simulink model "SerialWriteTriggeredSubsystem"  (R2018a)
settings: Solver=FixedStepAuto  StartTime=0.0  StopTime=10.0  FixedStep=.25  RelTol=1e-3  EnableMultiTasking=on
libraries: arduinolib x2
settings Model: ExtModeTrigDuration=2  Creator=jonathancoulter  LastModifiedBy=jonathancoulter
settings OptimizationCC: EnhancedBackFolding=on  PassReuseOutputArgsAs=Individual arguments  MaxStackSize=64  OptimizeBlockOrder=speed  DifferentSizesBufferReuse=on  OptimizationCustomize=off
settings DebuggingCC: ParameterTunabilityLossMsg=error
settings HardwareCC: ProdBitPerInt=16  ProdBitPerPointer=16  ProdBitPerSizeT=16  ProdBitPerPtrDiffT=16  ProdLargestAtomicFloat=None  ProdWordSize=8  ProdHWDeviceType=Atmel->AVR  UseEmbeddedCoderFeatures=off
settings SFSimCC: MATLABDynamicMemAlloc=off
settings RTWCC: SystemTargetFile=ert.tlc  HardwareBoard=Arduino Mega 2560  TLCOptions=-aInlineSetEventsForThisBaseRateFcn=TLC_FALSE -aSuppressMultiTaskScheduler=TLC_FALSE -aRateBasedStepFcn=1  TemplateMakefile=ert_default_tmf  Toolchain=Arduino AVR  BuildConfiguration=Faster Runs  IncludeHyperlinkInReport=on
settings CodeAppCC: ForceParamTrailComments=on  IgnoreCustomStorageClasses=off  OperatorAnnotations=on  SimulinkDataObjDesc=on  SFDataObjDesc=on  InsertBlockDesc=on
settings ERTTargetCC: SupportContinuousTime=on  SupportNonInlinedSFcns=on  SupportVariableSizeSignals=on

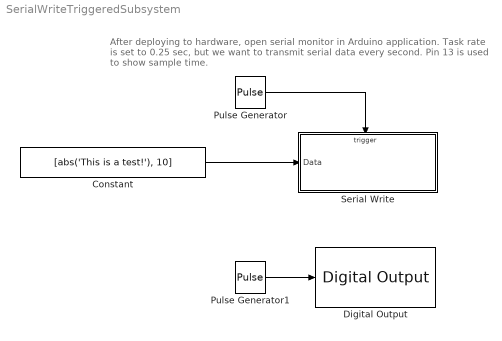
== system SerialWriteTriggeredSubsystem ==
  note: After deploying to hardware, open serial monitor in Arduino application.
      | Task rate is set to 0.25 sec, but we want to transmit serial data every second.
      | Pin 13 is used to show sample time.
  Constant : Constant  Value=[abs('This is a test!'), 10]
  Digital Output : arduinolib/Digital Output  pinNumber=13  blockPlatform=arduino
  Pulse Generator : DiscretePulseGenerator  Period=4  PulseWidth=2  SampleTime=-1
  Pulse Generator1 : DiscretePulseGenerator  SampleTime=-1
  Serial Write : Subsystem
  wires:
  Constant/1 -> Serial Write/1(Data)
  Pulse Generator/1 -> Serial Write/Trigger
  Pulse Generator1/1 -> Digital Output/1

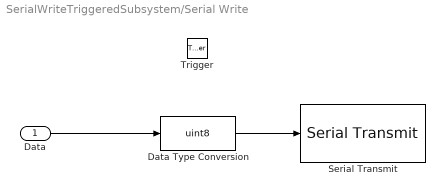
== system SerialWriteTriggeredSubsystem/Serial Write ==
  Data : Inport
  Trigger : TriggerPort  VariantControl=Variant  PortDimensions=1
  Data Type Conversion : DataTypeConversion  OutDataTypeStr=uint8
  Serial Transmit : arduinolib/Serial Transmit  portNumber=0  sendmode=write  sendformat=Decimal  floatprecision=2  blockPlatform=arduino
      settings: SourceProductName=Simulink Support Package for Arduino Hardware
  wires:
  Data/1 -> Data Type Conversion/1
  Data Type Conversion/1 -> Serial Transmit/1
